simulink model "exp5_9"  (Simulink 6.6)
settings: Solver=FixedStepDiscrete  SolverMode=SingleTasking  StartTime=0.0  StopTime=10.0  RelTol=1e-3  AbsTol=1e-6
settings Model: Creator=Administrator  LastModifiedBy=Administrator  ExtModeTrigMode=oneshot  ExtModeArmWhenConnect=off  ExtModeAutoUpdateStatusClock=off
settings DataIOCC: LimitDataPoints=off  TimeSaveName=t  OutputSaveName=y
settings OptimizationCC: BlockReduction=off  BooleanDataType=off
settings DebuggingCC: SignalResolutionControl=TryResolveAllWithWarning  SolverPrmCheckMsg=none  MultiTaskDSMMsg=warning  MultiTaskCondExecSysMsg=none  StrictBusMsg=None
settings HardwareCC: TargetUnknown=on
settings RTWCC: TemplateMakefile=grt_vc.tmf  IncludeERTFirstTime=on

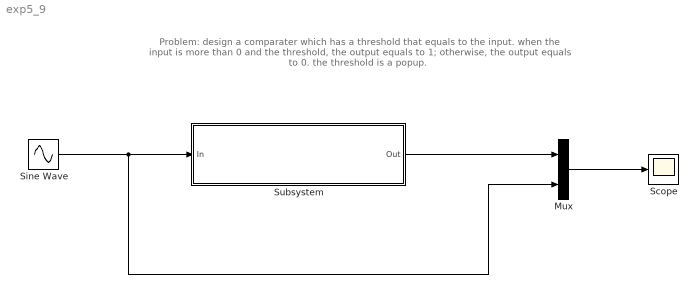
== system exp5_9 ==
  note: Problem: design a comparater which has a threshold that equals to the input.
      | when the input is more than 0 and the threshold, the output equals to 1; otherwise, the output equals to 0.
      | the threshold is a popup.
  Mux : Mux  Inputs=2
  Scope : Scope
      settings: TickLabels=on  TimeRange=10  DataFormat=Array
  Sine Wave : Sin  Amplitude=5  SampleTime=0
  Subsystem : Subsystem  mask(comparater){th=0.3}
      mask prompts: th "threshold"
      mask StyleString: popup(0.1|0.2|0.3)
      mask Display: disp('The Comparater')
  wires:
  Subsystem/1(Out) -> Mux/1
  Mux/1 -> Scope/1
  Sine Wave/1 -> Subsystem/1(In), Mux/2

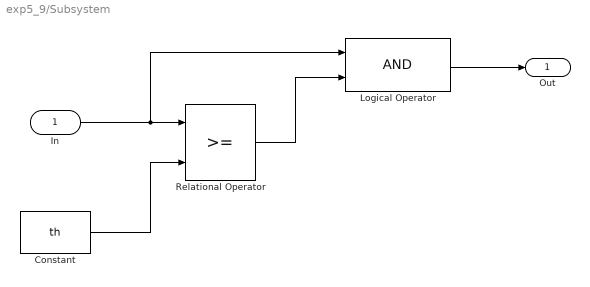
== system exp5_9/Subsystem ==
  In : Inport
  Constant : Constant  Value=th
  Logical Operator : Logic
  Relational Operator : RelationalOperator  InputSameDT=on
  Out : Outport  InitialOutput=0
  wires:
  Logical Operator/1 -> Out/1
  In/1 -> Logical Operator/1, Relational Operator/1
  Constant/1 -> Relational Operator/2
  Relational Operator/1 -> Logical Operator/2
